simulink model "wheel_leg"  (R2025b)
settings: Solver=VariableStepAuto  StartTime=0.0  StopTime=10  FixedStep=0.0001  RelTol=1e-3
values from neighbouring files (symbols this model uses):
  g = 9.8    [part1_dynamic.m]    (also in simulation.m)
  M_L_support = 1.44/2 + 0.045*2    (= 0.81)    [part1_dynamic.m]
  N = length(x_uniform)    [sweep_Ncut.m]
  N_filter = results(i).N    [sweep_Ncut.m]
  X = [theta; dtheta; x; dx; phi; dphi]    [part1_dynamic.m]    (also in simulation.m)
  Y = fft(x_uniform)    [sweep_Ncut.m]
undefined symbols (not defined in the file or in its folder): KD_leg, KP_leg, Z
libraries: sm_lib x76, nesl_utility x20, slpidlib x4
(part 3 of 3)

== matlab function wheel_leg/MATLAB Function11 ==
  data: phi1 input; T1 output; phi4 input; F_command input; Tp input; T4 output
function [T1,T4] = simcall_fivebar_vmc_torque_func(phi1,phi4,F_command,Tp)

    [T1,T4] = fivebar_vmc_torque_func(phi1,phi4,F_command,Tp);
    
end

== matlab function wheel_leg/MATLAB Function6 ==
  data: pai1 input; L0 output; pai0 output; pai4 input
function [L0,pai0] = simcall_fivebar_kinematics_func(pai1,pai4)

[L0,pai0] = fivebar_kinematics_func(pai1,pai4);

== matlab function wheel_leg/MATLAB Function7 ==
  data: L0 input; K output
function K = simcall_get_k_cubic_length(L0)

K = zeros(2,6);              % 明确告诉 Simulink：K 是 2×6
K(:,:) = get_k_cubic_length(L0);

end

== matlab function wheel_leg/MATLAB Function8 ==
  data: K input; theta input; T output; dtheta input; x input; Tp output; dx input; phi input; dphi input; theta_d input; dtheta_d input; x_d input; dx_d input; phi_d input; dphi_d input
function [T,Tp] = Get_U(K, theta, dtheta, x, dx, phi, dphi, ...
                                          theta_d, dtheta_d, x_d, dx_d, phi_d, dphi_d)
   
    X = [
        theta;
        dtheta;
        x;
        dx;
        phi;
        dphi
    ];
    
    Xd = [
        theta_d;
        dtheta_d;
        x_d;
        dx_d;
        phi_d;
        dphi_d
    ];
    U = -K*(X - Xd);
    T = U(1);
    Tp = U(2);
end

== matlab function wheel_leg/MATLAB Function9 ==
  data: phi1 input; dL0 output; phi4 input; dphi1 input; dphi4 input; dphi0 output
function [dL0,dphi0] = simcall_fivebar_velocity_func(phi1,phi4,dphi1,dphi4)

[dL0,dphi0] = fivebar_velocity_func(phi1,phi4,dphi1,dphi4);

end

== matlab function wheel_leg/MATLAB Function12 ==
  data: fn input; KP_theta output; zeta input; L_L0 input; R_L0 input; KD_theta output
function [KP_theta, KD_theta] = simcall_calc_fai0_diff_PD(fn, zeta, L_L0, R_L0)

[KP_theta, KD_theta] = calc_fai0_diff_PD(fn, zeta, L_L0, R_L0);
end

== matlab function wheel_leg/MATLAB Function13 ==
  data: tau_yaw input; KP_yaw_rate output; r_w input; Iz output
function [KP_yaw_rate, Iz] = simcall_calc_yaw_KP_tau(tau_yaw, r_w)
 [KP_yaw_rate, Iz] = calc_yaw_KP_tau(tau_yaw, r_w);
end

== matlab function wheel_leg/MATLAB Function1 ==
  data: L0 input; K output
function K = simcall_get_k_cubic_length(L0)

K = zeros(2,6);              % 明确告诉 Simulink：K 是 2×6
K(:,:) = get_k_cubic_length(L0);

end

== matlab function wheel_leg/MATLAB Function ==
  data: pai1 input; L0 output; pai0 output; pai4 input
function [L0,pai0] = simcall_fivebar_kinematics_func(pai1,pai4)

[L0,pai0] = fivebar_kinematics_func(pai1,pai4);

== matlab function wheel_leg/MATLAB Function2 ==
  data: K input; theta input; T output; dtheta input; x input; Tp output; dx input; phi input; dphi input; theta_d input; dtheta_d input; x_d input; dx_d input; phi_d input; dphi_d input
function [T,Tp] = Get_U(K, theta, dtheta, x, dx, phi, dphi, ...
                                          theta_d, dtheta_d, x_d, dx_d, phi_d, dphi_d)
   
    X = [
        theta;
        dtheta;
        x;
        dx;
        phi;
        dphi
    ];
    
    Xd = [
        theta_d;
        dtheta_d;
        x_d;
        dx_d;
        phi_d;
        dphi_d
    ];
    U = -K*(X - Xd);
    T = U(1);
    Tp = U(2);
end

== matlab function wheel_leg/MATLAB Function3 ==
  data: phi1 input; dL0 output; phi4 input; dphi1 input; dphi4 input; dphi0 output
function [dL0,dphi0] = simcall_fivebar_velocity_func(phi1,phi4,dphi1,dphi4)

[dL0,dphi0] = fivebar_velocity_func(phi1,phi4,dphi1,dphi4);

end

== matlab function wheel_leg/MATLAB Function4 ==
  data: phi0 input; theta output; dphi0 input; body_phi input; body_dphi input; dtheta output
function [theta,dtheta] = simcall_fivebar_theta_func(phi0,dphi0,body_phi,body_dphi)

    [theta,dtheta] = fivebar_theta_func(phi0,dphi0,body_phi,body_dphi);

end

== matlab function wheel_leg/MATLAB Function5 ==
  data: phi1 input; T1 output; phi4 input; F_command input; Tp input; T4 output
function [T1,T4] = simcall_fivebar_vmc_torque_func(phi1,phi4,F_command,Tp)

    [T1,T4] = fivebar_vmc_torque_func(phi1,phi4,F_command,Tp);
    
end

== matlab function wheel_leg/MATLAB Function10 ==
  data: phi0 input; theta output; dphi0 input; body_phi input; body_dphi input; dtheta output
function [theta,dtheta] = simcall_fivebar_theta_func(phi0,dphi0,body_phi,body_dphi)

    [theta,dtheta] = fivebar_theta_func(phi0,dphi0,body_phi,body_dphi);

end
